simulink model "DuckCarSim_ExpValues"  (R2023b)
settings: Solver=VariableStepAuto  StartTime=0.0  StopTime=10  MaxStep=0.001  RelTol=1e-3  EnableMultiTasking=on
values from neighbouring files (symbols this model uses):
  finalDistInch = 13.00    (= 13)    [DuckCarLab3.m]
  K_a = 1.2    [DuckCarLab3.m]
  K_m_inch = K_m/0.0254    [DuckCarLab3.m]
  K_p_damp = 2.942    [DuckCarLab3.m]
  K_p_sixNine = 6.84    [DuckCarLab3.m]
  nonLinearSensor = [0.0864192841833102 , 0.140817267512297]    [DuckCarLab3.m]
  standOffDistInch = 7.00    (= 7)    [DuckCarLab3.m]
  standoffV = 1.335    [DuckCarLab3.m]
undefined symbols (not defined in the file or in its folder): tau_xDamp, tau_xSixNine
settings Model: Creator=AllisonBT  LastModifiedBy=n8dsa
settings SolverCC: AlgebraicLoopSolver=TrustRegion
settings DataIOCC: ReturnWorkspaceOutputs=off
settings OptimizationCC: LifeSpan=inf
settings DebuggingCC: UnconnectedInputMsg=warning  UnconnectedOutputMsg=warning  UnconnectedLineMsg=warning  SFUnexpectedBacktrackingDiag=warning  SFNoUnconditionalDefaultTransitionDiag=warning  ArithmeticOperatorsInVariantConditions=warning
settings ModelReferenceCC: EnableRefExpFcnMdlSchedulingChecks=on
settings SFSimCC: SimUseLocalCustomCode=off  CustomCodeUndefinedFunction=UseInterfaceOnly
settings RTWCC: RTWUseLocalCustomCode=off
settings CodeAppCC: StateflowObjectComments=on
settings GRTTargetCC: TargetLangStandard=C89/C90 (ANSI)
settings ConfigComp: CovMetricSettings=dw  CovSaveCumulativeToWorkspaceVar=on  CovSaveSingleToWorkspaceVar=on  CovExternalEMLEnable=off

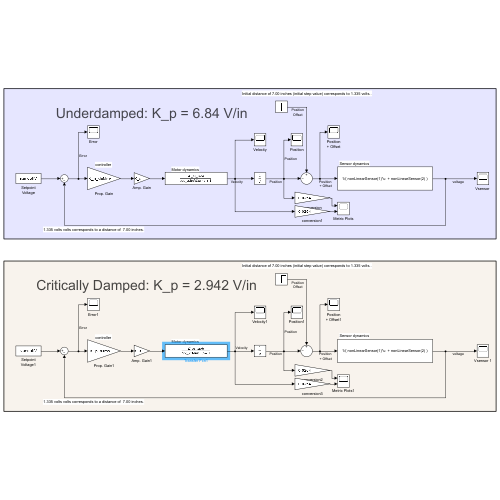
[thumbnail: Simulink's stored preview of the top-level diagram]
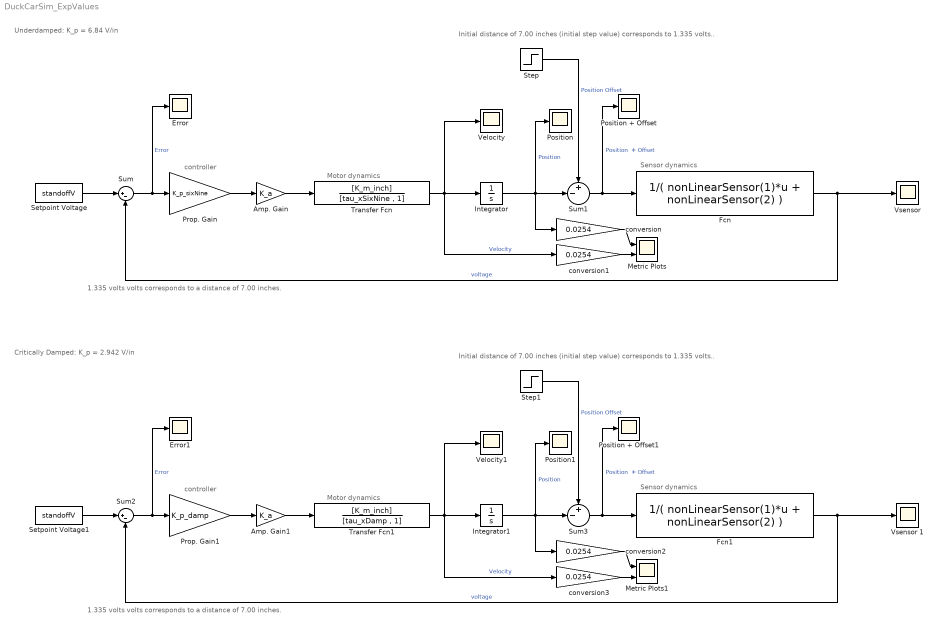
== system DuckCarSim_ExpValues ==
  note: Underdamped: K_p = 6.84 V/in
  note: Sensor dynamics
  note: Motor dynamics
  note: 1.335 volts volts corresponds to a distance of 7.00 inches.
  note: Initial distance of 7.00 inches (initial step value) corresponds to 1.335 volts..
  note: controller
  note: Critically Damped: K_p = 2.942 V/in
  note: Sensor dynamics
  note: Motor dynamics
  note: controller
  note: Initial distance of 7.00 inches (initial step value) corresponds to 1.335 volts..
  note: 1.335 volts volts corresponds to a distance of 7.00 inches.
  Amp. Gain : Gain  Gain=K_a
  Amp. Gain1 : Gain  Gain=K_a
  Error : Scope
  Error1 : Scope
  Fcn : Fcn  Expr="1/( nonLinearSensor(1)*u  + nonLinearSensor(2) )"
  Fcn1 : Fcn  Expr="1/( nonLinearSensor(1)*u  + nonLinearSensor(2) )"
  Integrator : Integrator
  Integrator1 : Integrator
  Metric Plots : Scope  NumInputPorts=2
  Metric Plots1 : Scope  NumInputPorts=2
  Position : Scope
  Position + Offset : Scope
  Position + Offset1 : Scope
  Position1 : Scope
  Prop. Gain : Gain  Gain=K_p_sixNine
  Prop. Gain1 : Gain  Gain=K_p_damp
  Setpoint Voltage : Constant  Value=standoffV
  Setpoint Voltage1 : Constant  Value=standoffV
  Step : Step  Time=0  Before=standOffDistInch  After=finalDistInch  SampleTime=0
  Step1 : Step  Time=0  Before=standOffDistInch  After=finalDistInch  SampleTime=0
  Sum : Sum  Inputs=|+-
  Sum1 : Sum  Inputs=+-|
  Sum2 : Sum  Inputs=|+-
  Sum3 : Sum  Inputs=+-|
  Transfer Fcn : TransferFcn  Numerator=[K_m_inch]  Denominator=[tau_xSixNine , 1]
  Transfer Fcn1 : TransferFcn  Numerator=[K_m_inch]  Denominator=[tau_xDamp , 1]
  Velocity : Scope
  Velocity1 : Scope
  "Vsensor " : Scope
  Vsensor 1 : Scope
  conversion{,1..3} (4 alike) : Gain  Gain=0.0254
  wires:
  Amp. Gain/1 -> Transfer Fcn/1
  Prop. Gain/1 -> Amp. Gain/1
  Sum/1 -> Error/1, Prop. Gain/1  "Error"
  Fcn/1 -> Sum/2, "Vsensor "/1  "voltage"
  Setpoint Voltage/1 -> Sum/1
  Transfer Fcn/1 -> conversion1/1, Integrator/1, Velocity/1  "Velocity"
  Step/1 -> Sum1/1  "Position Offset"
  Sum1/1 -> Position + Offset/1, Fcn/1  "Position  + Offset"
  Integrator/1 -> conversion/1, Position/1, Sum1/2  "Position"
  conversion/1 -> Metric Plots/1
  conversion1/1 -> Metric Plots/2
  Prop. Gain1/1 -> Amp. Gain1/1
  Step1/1 -> Sum3/1  "Position Offset"
  Sum2/1 -> Error1/1, Prop. Gain1/1  "Error"
  Amp. Gain1/1 -> Transfer Fcn1/1
  Integrator1/1 -> conversion2/1, Position1/1, Sum3/2  "Position"
  Transfer Fcn1/1 -> conversion3/1, Integrator1/1, Velocity1/1  "Velocity"
  Sum3/1 -> Position + Offset1/1, Fcn1/1  "Position  + Offset"
  conversion2/1 -> Metric Plots1/1
  conversion3/1 -> Metric Plots1/2
  Setpoint Voltage1/1 -> Sum2/1
  Fcn1/1 -> Sum2/2, Vsensor 1/1  "voltage"
